simulink model "prob_1a"  (R2020a)
settings: Solver=VariableStepAuto  StartTime=0.0  StopTime=10.0  RelTol=1e-3
values from neighbouring files (symbols this model uses):
  J = 2000    [params.m]
  Kd = 2 * zeta * sqrt(Kp * J)    [params.m]
  Kp = J * wn^2    (= 18000)    [params.m]
settings Model: Creator=VTOL_HYD  LastModifiedBy=VTOL_HYD

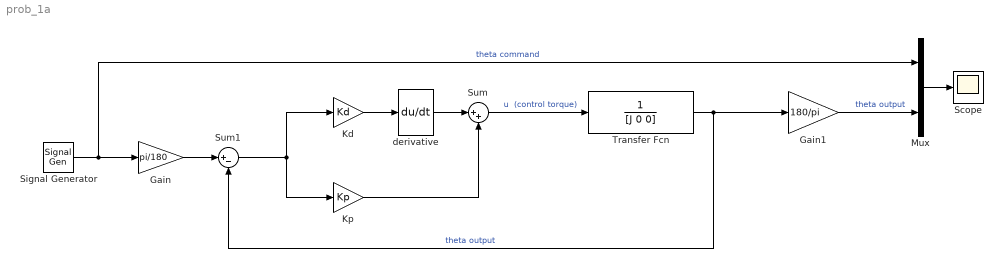
== system prob_1a ==
  Gain : Gain  Gain=pi/180
  Gain1 : Gain  Gain=180/pi
  Kd : Gain  Gain=Kd
  Kp : Gain  Gain=Kp
  Mux : Mux  Inputs=2
  Scope : Scope
  Signal Generator : SignalGenerator  WaveForm=square  Amplitude=30  Units=rad/sec
  Sum : Sum  Inputs=|++
  Sum1 : Sum  Inputs=|+-
  Transfer Fcn : TransferFcn  Denominator=[J 0 0]
  derivative : Derivative
  wires:
  Kd/1 -> derivative/1
  derivative/1 -> Sum/1
  Kp/1 -> Sum/2
  Sum/1 -> Transfer Fcn/1  "u  (control torque)"
  Transfer Fcn/1 -> Gain1/1, Sum1/2  "theta output"
  Sum1/1 -> Kp/1, Kd/1
  Signal Generator/1 -> Mux/1, Gain/1  "theta command"
  Gain/1 -> Sum1/1
  Gain1/1 -> Mux/2  "theta output"
  Mux/1 -> Scope/1
